simulink model "T1_PreLab_2"  (R2023a)
settings: Solver=VariableStepAuto  StartTime=0.0  StopTime=100  RelTol=1e-3
libraries: dspmathops x30, dspfdesign x15, dspsrcs4 x15, commsink2 x15, dspsigops x15, commrandsrc3 x1
settings Model: Creator=HP VICTUS  LastModifiedBy=HP VICTUS

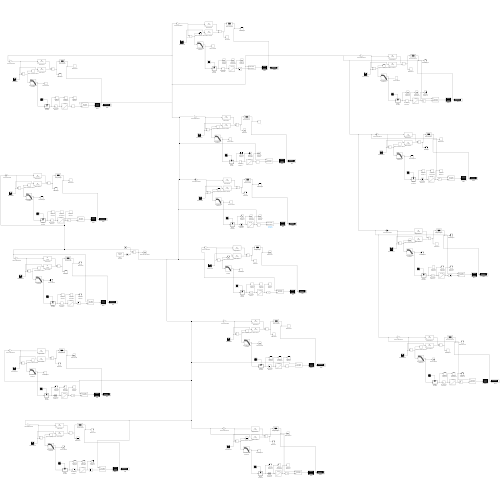
[thumbnail: Simulink's stored preview of the top-level diagram]
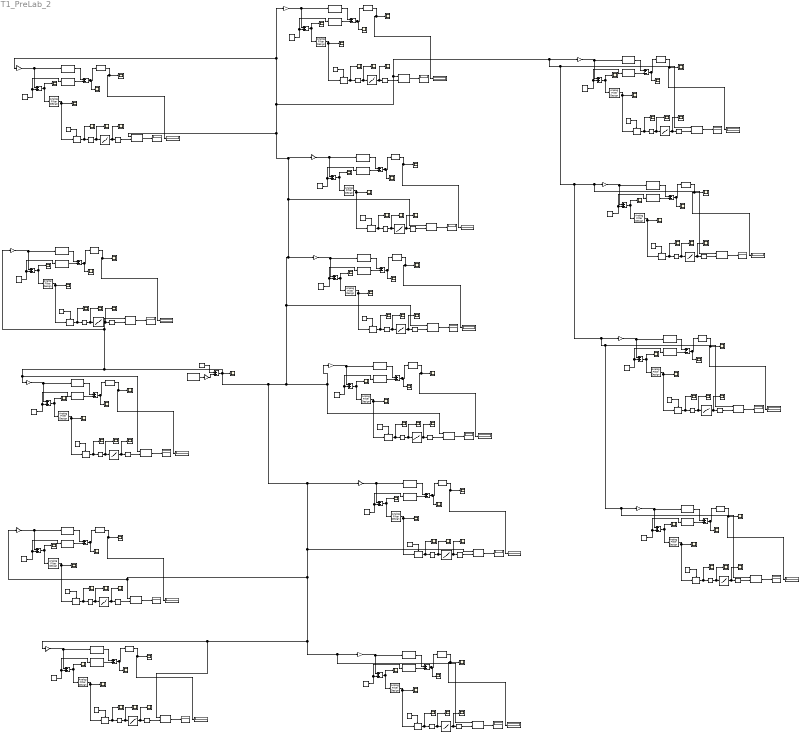
== system T1_PreLab_2 ==
  1-D Lookup Table{,1..14} (15 alike) : Lookup_n-D  NumberOfTableDimensions=1  BreakpointsForDimension1=[-1,1]  Table=[-4,4]  TableDataTypeStr=Inherit: Inherit from 'Table data'  InternalRulePriority=Speed  RndMeth=Simplest
  Add{,1..15} (16 alike) : Sum
  BER{,1..14} (15 alike) : Display
  Binary Generator : commrandsrc3/Bernoulli Binary Generator  ProbabilityOfZero=0.5  SeedSource=Parameter  Seed=61  SampleTime=0.1  SamplesPerFrame=1  OutputDataType=double  SimulateUsing=Interpreted execution
  Channel Attenuation{,1..14} (15 alike) : Gain  Gain=0.5
  Channel Bandwidth Limitation{,1..14} (15 alike) : dspfdesign/Analog Filter Design  method=Butterworth  filttype=Lowpass  N=10  Wlo=1000  Whi=80  Rp=2  Rs=40
  Channel Noise : dspsrcs4/Random Source  SrcType=Gaussian  NormMethod=Ziggurat  CltLength=12  MinVal=0  MaxVal=1  MeanVal=0  VarVal=2  RepMode=Not repeatable  rawSeed=1  IsInherit=off  SampMode=Discrete  SampTime=0.01  SampFrame=1  DataType=Double  OutComplex=Real  OutputFrames=off
  Channel Noise1 : dspsrcs4/Random Source  SrcType=Gaussian  NormMethod=Ziggurat  CltLength=12  MinVal=0  MaxVal=1  MeanVal=0  VarVal=1.6  RepMode=Not repeatable  rawSeed=1  IsInherit=off  SampMode=Discrete  SampTime=0.01  SampFrame=1  DataType=Double  OutComplex=Real  OutputFrames=off
  Channel Noise10 : dspsrcs4/Random Source  SrcType=Gaussian  NormMethod=Ziggurat  CltLength=12  MinVal=0  MaxVal=1  MeanVal=0  VarVal=2.8  RepMode=Not repeatable  rawSeed=1  IsInherit=off  SampMode=Discrete  SampTime=0.01  SampFrame=1  DataType=Double  OutComplex=Real  OutputFrames=off
  Channel Noise11 : dspsrcs4/Random Source  SrcType=Gaussian  NormMethod=Ziggurat  CltLength=12  MinVal=0  MaxVal=1  MeanVal=0  VarVal=2.3  RepMode=Not repeatable  rawSeed=1  IsInherit=off  SampMode=Discrete  SampTime=0.01  SampFrame=1  DataType=Double  OutComplex=Real  OutputFrames=off
  Channel Noise12 : dspsrcs4/Random Source  SrcType=Gaussian  NormMethod=Ziggurat  CltLength=12  MinVal=0  MaxVal=1  MeanVal=0  VarVal=3.5  RepMode=Not repeatable  rawSeed=1  IsInherit=off  SampMode=Discrete  SampTime=0.01  SampFrame=1  DataType=Double  OutComplex=Real  OutputFrames=off
  Channel Noise13 : dspsrcs4/Random Source  SrcType=Gaussian  NormMethod=Ziggurat  CltLength=12  MinVal=0  MaxVal=1  MeanVal=0  VarVal=0.2  RepMode=Not repeatable  rawSeed=1  IsInherit=off  SampMode=Discrete  SampTime=0.01  SampFrame=1  DataType=Double  OutComplex=Real  OutputFrames=off
  Channel Noise14 : dspsrcs4/Random Source  SrcType=Gaussian  NormMethod=Ziggurat  CltLength=12  MinVal=0  MaxVal=1  MeanVal=0  VarVal=0.4  RepMode=Not repeatable  rawSeed=1  IsInherit=off  SampMode=Discrete  SampTime=0.01  SampFrame=1  DataType=Double  OutComplex=Real  OutputFrames=off
  Channel Noise2 : dspsrcs4/Random Source  SrcType=Gaussian  NormMethod=Ziggurat  CltLength=12  MinVal=0  MaxVal=1  MeanVal=0  VarVal=1.9  RepMode=Not repeatable  rawSeed=1  IsInherit=off  SampMode=Discrete  SampTime=0.01  SampFrame=1  DataType=Double  OutComplex=Real  OutputFrames=off
  Channel Noise3 : dspsrcs4/Random Source  SrcType=Gaussian  NormMethod=Ziggurat  CltLength=12  MinVal=0  MaxVal=1  MeanVal=0  VarVal=2.4  RepMode=Not repeatable  rawSeed=1  IsInherit=off  SampMode=Discrete  SampTime=0.01  SampFrame=1  DataType=Double  OutComplex=Real  OutputFrames=off
  Channel Noise4 : dspsrcs4/Random Source  SrcType=Gaussian  NormMethod=Ziggurat  CltLength=12  MinVal=0  MaxVal=1  MeanVal=0  VarVal=0.3  RepMode=Not repeatable  rawSeed=1  IsInherit=off  SampMode=Discrete  SampTime=0.01  SampFrame=1  DataType=Double  OutComplex=Real  OutputFrames=off
  Channel Noise5 : dspsrcs4/Random Source  SrcType=Gaussian  NormMethod=Ziggurat  CltLength=12  MinVal=0  MaxVal=1  MeanVal=0  VarVal=0.5  RepMode=Not repeatable  rawSeed=1  IsInherit=off  SampMode=Discrete  SampTime=0.01  SampFrame=1  DataType=Double  OutComplex=Real  OutputFrames=off
  Channel Noise6 : dspsrcs4/Random Source  SrcType=Gaussian  NormMethod=Ziggurat  CltLength=12  MinVal=0  MaxVal=1  MeanVal=0  VarVal=0.7  RepMode=Not repeatable  rawSeed=1  IsInherit=off  SampMode=Discrete  SampTime=0.01  SampFrame=1  DataType=Double  OutComplex=Real  OutputFrames=off
  Channel Noise7 : dspsrcs4/Random Source  SrcType=Gaussian  NormMethod=Ziggurat  CltLength=12  MinVal=0  MaxVal=1  MeanVal=0  VarVal=0.1  RepMode=Not repeatable  rawSeed=1  IsInherit=off  SampMode=Discrete  SampTime=0.01  SampFrame=1  DataType=Double  OutComplex=Real  OutputFrames=off
  Channel Noise8 : dspsrcs4/Random Source  SrcType=Gaussian  NormMethod=Ziggurat  CltLength=12  MinVal=0  MaxVal=1  MeanVal=0  VarVal=1.3  RepMode=Not repeatable  rawSeed=1  IsInherit=off  SampMode=Discrete  SampTime=0.01  SampFrame=1  DataType=Double  OutComplex=Real  OutputFrames=off
  Channel Noise9 : dspsrcs4/Random Source  SrcType=Gaussian  NormMethod=Ziggurat  CltLength=12  MinVal=0  MaxVal=1  MeanVal=0  VarVal=1  RepMode=Not repeatable  rawSeed=1  IsInherit=off  SampMode=Discrete  SampTime=0.01  SampFrame=1  DataType=Double  OutComplex=Real  OutputFrames=off
  Channel Output{,1..14} (15 alike) : Scope
  Constant : Constant  Value=-4  SampleTime=-1
  Digital Information Signal : Scope
  Error Rate Calculation{,1..14} (15 alike) : commsink2/Error Rate Calculation  N=1  st_delay=0  cp_mode=Entire frame  subframe=[]  PMode=Port  WsName=ErrorVec  RsMode2=off  stop=off  numErr=100  maxBits=1e6
      settings: LibrarySourceBlock=|
      | commhdlsink/Error Rate
      | Calculation
  Gain : Gain  Gain=8
  Moving Average{,1..14} (15 alike) : DiscreteFir  Coefficients=ones(1,1000)/1000  SampleTime=0.001
  Noise  Power{,1..14} (15 alike) : dspmathops/dB Conversion  dBtype=dB  intype=Amplitude  R=1  fuzz=off
      settings: LibrarySourceBlock=commutil2/dB Conversion
  Output from Detector{,1..14} (15 alike) : Scope
  Output from Sampler{,1..14} (15 alike) : Scope
  Output from Thresholder{,1..14} (15 alike) : Scope
  Pulse Generator{,1..14} (15 alike) : DiscretePulseGenerator  PulseType=Time based  Period=0.1  PulseWidth=50
  SNR{,1..14} (15 alike) : Display
  SNR Average{,1..14} (15 alike) : Scope
  SNR Graph{,1..14} (15 alike) : Scope
  Sample and Hold{,1..14} (15 alike) : dspsigops/Sample and Hold  trig=Rising edge  initCond=0  latchinput=off
  Signal Power{,1..14} (15 alike) : dspmathops/dB Conversion  dBtype=dB  intype=Amplitude  R=1  fuzz=off
      settings: LibrarySourceBlock=commutil2/dB Conversion
  Signal corrupted by Noice{,1..14} (15 alike) : Scope
  Subtract{,1..14} (15 alike) : Sum  Inputs=+-
  Zero Crossing Detector{,1..14} (15 alike) : Signum
  Zero-Order Hold{,1..14} (15 alike) : ZeroOrderHold  SampleTime=0.1
  wires:
  Binary Generator/1 -> Gain/1
  Gain/1 -> Add/2
  Constant/1 -> Add/1
  Channel Attenuation/1 -> Add1/1, Signal Power/1
  Channel Noise/1 -> Add1/2, Noise  Power/1
  Add1/1 -> Channel Bandwidth Limitation/1, Signal corrupted by Noice/1
  Channel Bandwidth Limitation/1 -> Sample and Hold/1, Channel Output/1
  Pulse Generator/1 -> Sample and Hold/Trigger
  Error Rate Calculation/1 -> BER/1
  Zero-Order Hold/1 -> Error Rate Calculation/2
  1-D Lookup Table/1 -> Output from Detector/1, Zero-Order Hold/1
  Zero Crossing Detector/1 -> Output from Thresholder/1, 1-D Lookup Table/1
  Sample and Hold/1 -> Output from Sampler/1, Zero Crossing Detector/1
  Moving Average/1 -> SNR/1, SNR Average/1
  Subtract/1 -> SNR Graph/1, Moving Average/1
  Signal Power/1 -> Subtract/1
  Noise  Power/1 -> Subtract/2
  Noise  Power1/1 -> Subtract1/2
  Subtract1/1 -> SNR Graph1/1, Moving Average1/1
  Sample and Hold1/1 -> Output from Sampler1/1, Zero Crossing Detector1/1
  Signal Power1/1 -> Subtract1/1
  Error Rate Calculation1/1 -> BER1/1
  Zero-Order Hold1/1 -> Error Rate Calculation1/2
  Channel Bandwidth Limitation1/1 -> Sample and Hold1/1, Channel Output1/1
  Add2/1 -> Channel Bandwidth Limitation1/1, Signal corrupted by Noice1/1
  Moving Average1/1 -> SNR1/1, SNR Average1/1
  Pulse Generator1/1 -> Sample and Hold1/Trigger
  Channel Attenuation1/1 -> Add2/1, Signal Power1/1
  Channel Noise1/1 -> Add2/2, Noise  Power1/1
  Zero Crossing Detector1/1 -> Output from Thresholder1/1, 1-D Lookup Table1/1
  1-D Lookup Table1/1 -> Output from Detector1/1, Zero-Order Hold1/1
  Noise  Power2/1 -> Subtract2/2
  Subtract2/1 -> SNR Graph2/1, Moving Average2/1
  Sample and Hold2/1 -> Output from Sampler2/1, Zero Crossing Detector2/1
  Signal Power2/1 -> Subtract2/1
  Error Rate Calculation2/1 -> BER2/1
  Zero-Order Hold2/1 -> Error Rate Calculation2/2
  Channel Bandwidth Limitation2/1 -> Sample and Hold2/1, Channel Output2/1
  Add3/1 -> Channel Bandwidth Limitation2/1, Signal corrupted by Noice2/1
  Moving Average2/1 -> SNR2/1, SNR Average2/1
  Pulse Generator2/1 -> Sample and Hold2/Trigger
  Channel Attenuation2/1 -> Add3/1, Signal Power2/1
  Channel Noise2/1 -> Add3/2, Noise  Power2/1
  Zero Crossing Detector2/1 -> Output from Thresholder2/1, 1-D Lookup Table2/1
  1-D Lookup Table2/1 -> Output from Detector2/1, Zero-Order Hold2/1
  Noise  Power3/1 -> Subtract3/2
  Subtract3/1 -> SNR Graph3/1, Moving Average3/1
  Sample and Hold3/1 -> Output from Sampler3/1, Zero Crossing Detector3/1
  Signal Power3/1 -> Subtract3/1
  Error Rate Calculation3/1 -> BER3/1
  Zero-Order Hold3/1 -> Error Rate Calculation3/2
  Channel Bandwidth Limitation3/1 -> Sample and Hold3/1, Channel Output3/1
  Add4/1 -> Channel Bandwidth Limitation3/1, Signal corrupted by Noice3/1
  Moving Average3/1 -> SNR3/1, SNR Average3/1
  Pulse Generator3/1 -> Sample and Hold3/Trigger
  Channel Attenuation3/1 -> Add4/1, Signal Power3/1
  Channel Noise3/1 -> Add4/2, Noise  Power3/1
  Zero Crossing Detector3/1 -> Output from Thresholder3/1, 1-D Lookup Table3/1
  1-D Lookup Table3/1 -> Output from Detector3/1, Zero-Order Hold3/1
  Noise  Power4/1 -> Subtract4/2
  Subtract4/1 -> SNR Graph4/1, Moving Average4/1
  Sample and Hold4/1 -> Output from Sampler4/1, Zero Crossing Detector4/1
  Signal Power4/1 -> Subtract4/1
  Error Rate Calculation4/1 -> BER4/1
  Zero-Order Hold4/1 -> Error Rate Calculation4/2
  Channel Bandwidth Limitation4/1 -> Sample and Hold4/1, Channel Output4/1
  Add5/1 -> Channel Bandwidth Limitation4/1, Signal corrupted by Noice4/1
  Moving Average4/1 -> SNR4/1, SNR Average4/1
  Pulse Generator4/1 -> Sample and Hold4/Trigger
  Channel Attenuation4/1 -> Add5/1, Signal Power4/1
  Channel Noise4/1 -> Add5/2, Noise  Power4/1
  Zero Crossing Detector4/1 -> Output from Thresholder4/1, 1-D Lookup Table4/1
  1-D Lookup Table4/1 -> Output from Detector4/1, Zero-Order Hold4/1
  Noise  Power5/1 -> Subtract5/2
  Subtract5/1 -> SNR Graph5/1, Moving Average5/1
  Sample and Hold5/1 -> Output from Sampler5/1, Zero Crossing Detector5/1
  Signal Power5/1 -> Subtract5/1
  Error Rate Calculation5/1 -> BER5/1
  Zero-Order Hold5/1 -> Error Rate Calculation5/2
  Channel Bandwidth Limitation5/1 -> Sample and Hold5/1, Channel Output5/1
  Add6/1 -> Channel Bandwidth Limitation5/1, Signal corrupted by Noice5/1
  Moving Average5/1 -> SNR5/1, SNR Average5/1
  Pulse Generator5/1 -> Sample and Hold5/Trigger
  Channel Attenuation5/1 -> Add6/1, Signal Power5/1
  Channel Noise5/1 -> Add6/2, Noise  Power5/1
  Zero Crossing Detector5/1 -> Output from Thresholder5/1, 1-D Lookup Table5/1
  1-D Lookup Table5/1 -> Output from Detector5/1, Zero-Order Hold5/1
  Noise  Power6/1 -> Subtract6/2
  Subtract6/1 -> SNR Graph6/1, Moving Average6/1
  Sample and Hold6/1 -> Output from Sampler6/1, Zero Crossing Detector6/1
  Signal Power6/1 -> Subtract6/1
  Error Rate Calculation6/1 -> BER6/1
  Zero-Order Hold6/1 -> Error Rate Calculation6/2
  Channel Bandwidth Limitation6/1 -> Sample and Hold6/1, Channel Output6/1
  Add7/1 -> Channel Bandwidth Limitation6/1, Signal corrupted by Noice6/1
  Moving Average6/1 -> SNR6/1, SNR Average6/1
  Pulse Generator6/1 -> Sample and Hold6/Trigger
  Channel Attenuation6/1 -> Add7/1, Signal Power6/1
  Channel Noise6/1 -> Add7/2, Noise  Power6/1
  Zero Crossing Detector6/1 -> Output from Thresholder6/1, 1-D Lookup Table6/1
  1-D Lookup Table6/1 -> Output from Detector6/1, Zero-Order Hold6/1
  Noise  Power7/1 -> Subtract7/2
  Subtract7/1 -> SNR Graph7/1, Moving Average7/1
  Sample and Hold7/1 -> Output from Sampler7/1, Zero Crossing Detector7/1
  Signal Power7/1 -> Subtract7/1
  Error Rate Calculation7/1 -> BER7/1
  Zero-Order Hold7/1 -> Error Rate Calculation7/2
  Channel Bandwidth Limitation7/1 -> Sample and Hold7/1, Channel Output7/1
  Add8/1 -> Channel Bandwidth Limitation7/1, Signal corrupted by Noice7/1
  Moving Average7/1 -> SNR7/1, SNR Average7/1
  Pulse Generator7/1 -> Sample and Hold7/Trigger
  Channel Attenuation7/1 -> Add8/1, Signal Power7/1
  Channel Noise7/1 -> Add8/2, Noise  Power7/1
  Zero Crossing Detector7/1 -> Output from Thresholder7/1, 1-D Lookup Table7/1
  1-D Lookup Table7/1 -> Output from Detector7/1, Zero-Order Hold7/1
  Noise  Power8/1 -> Subtract8/2
  Subtract8/1 -> SNR Graph8/1, Moving Average8/1
  Sample and Hold8/1 -> Output from Sampler8/1, Zero Crossing Detector8/1
  Signal Power8/1 -> Subtract8/1
  Error Rate Calculation8/1 -> BER8/1
  Zero-Order Hold8/1 -> Error Rate Calculation8/2
  Channel Bandwidth Limitation8/1 -> Sample and Hold8/1, Channel Output8/1
  Add9/1 -> Channel Bandwidth Limitation8/1, Signal corrupted by Noice8/1
  Moving Average8/1 -> SNR8/1, SNR Average8/1
  Pulse Generator8/1 -> Sample and Hold8/Trigger
  Channel Attenuation8/1 -> Add9/1, Signal Power8/1
  Channel Noise8/1 -> Add9/2, Noise  Power8/1
  Zero Crossing Detector8/1 -> Output from Thresholder8/1, 1-D Lookup Table8/1
  1-D Lookup Table8/1 -> Output from Detector8/1, Zero-Order Hold8/1
  Noise  Power9/1 -> Subtract9/2
  Subtract9/1 -> SNR Graph9/1, Moving Average9/1
  Sample and Hold9/1 -> Output from Sampler9/1, Zero Crossing Detector9/1
  Signal Power9/1 -> Subtract9/1
  Error Rate Calculation9/1 -> BER9/1
  Zero-Order Hold9/1 -> Error Rate Calculation9/2
  Channel Bandwidth Limitation9/1 -> Sample and Hold9/1, Channel Output9/1
  Add10/1 -> Channel Bandwidth Limitation9/1, Signal corrupted by Noice9/1
  Moving Average9/1 -> SNR9/1, SNR Average9/1
  Pulse Generator9/1 -> Sample and Hold9/Trigger
  Channel Attenuation9/1 -> Add10/1, Signal Power9/1
  Channel Noise9/1 -> Add10/2, Noise  Power9/1
  Zero Crossing Detector9/1 -> Output from Thresholder9/1, 1-D Lookup Table9/1
  1-D Lookup Table9/1 -> Output from Detector9/1, Zero-Order Hold9/1
  Noise  Power10/1 -> Subtract10/2
  Subtract10/1 -> SNR Graph10/1, Moving Average10/1
  Sample and Hold10/1 -> Output from Sampler10/1, Zero Crossing Detector10/1
  Signal Power10/1 -> Subtract10/1
  Error Rate Calculation10/1 -> BER10/1
  Zero-Order Hold10/1 -> Error Rate Calculation10/2
  Channel Bandwidth Limitation10/1 -> Sample and Hold10/1, Channel Output10/1
  Add11/1 -> Channel Bandwidth Limitation10/1, Signal corrupted by Noice10/1
  Moving Average10/1 -> SNR10/1, SNR Average10/1
  Pulse Generator10/1 -> Sample and Hold10/Trigger
  Channel Attenuation10/1 -> Add11/1, Signal Power10/1
  Channel Noise10/1 -> Add11/2, Noise  Power10/1
  Zero Crossing Detector10/1 -> Output from Thresholder10/1, 1-D Lookup Table10/1
  1-D Lookup Table10/1 -> Output from Detector10/1, Zero-Order Hold10/1
  Noise  Power11/1 -> Subtract11/2
  Subtract11/1 -> SNR Graph11/1, Moving Average11/1
  Sample and Hold11/1 -> Output from Sampler11/1, Zero Crossing Detector11/1
  Signal Power11/1 -> Subtract11/1
  Error Rate Calculation11/1 -> BER11/1
  Zero-Order Hold11/1 -> Error Rate Calculation11/2
  Channel Bandwidth Limitation11/1 -> Sample and Hold11/1, Channel Output11/1
  Add12/1 -> Channel Bandwidth Limitation11/1, Signal corrupted by Noice11/1
  Moving Average11/1 -> SNR11/1, SNR Average11/1
  Pulse Generator11/1 -> Sample and Hold11/Trigger
  Channel Attenuation11/1 -> Add12/1, Signal Power11/1
  Channel Noise11/1 -> Add12/2, Noise  Power11/1
  Zero Crossing Detector11/1 -> Output from Thresholder11/1, 1-D Lookup Table11/1
  1-D Lookup Table11/1 -> Output from Detector11/1, Zero-Order Hold11/1
  Noise  Power12/1 -> Subtract12/2
  Subtract12/1 -> SNR Graph12/1, Moving Average12/1
  Sample and Hold12/1 -> Output from Sampler12/1, Zero Crossing Detector12/1
  Signal Power12/1 -> Subtract12/1
  Error Rate Calculation12/1 -> BER12/1
  Zero-Order Hold12/1 -> Error Rate Calculation12/2
  Channel Bandwidth Limitation12/1 -> Sample and Hold12/1, Channel Output12/1
  Add13/1 -> Channel Bandwidth Limitation12/1, Signal corrupted by Noice12/1
  Moving Average12/1 -> SNR12/1, SNR Average12/1
  Pulse Generator12/1 -> Sample and Hold12/Trigger
  Channel Attenuation12/1 -> Add13/1, Signal Power12/1
  Channel Noise12/1 -> Add13/2, Noise  Power12/1
  Zero Crossing Detector12/1 -> Output from Thresholder12/1, 1-D Lookup Table12/1
  1-D Lookup Table12/1 -> Output from Detector12/1, Zero-Order Hold12/1
  Noise  Power13/1 -> Subtract13/2
  Subtract13/1 -> SNR Graph13/1, Moving Average13/1
  Sample and Hold13/1 -> Output from Sampler13/1, Zero Crossing Detector13/1
  Signal Power13/1 -> Subtract13/1
  Error Rate Calculation13/1 -> BER13/1
  Zero-Order Hold13/1 -> Error Rate Calculation13/2
  Channel Bandwidth Limitation13/1 -> Sample and Hold13/1, Channel Output13/1
  Add14/1 -> Channel Bandwidth Limitation13/1, Signal corrupted by Noice13/1
  Moving Average13/1 -> SNR13/1, SNR Average13/1
  Pulse Generator13/1 -> Sample and Hold13/Trigger
  Channel Attenuation13/1 -> Add14/1, Signal Power13/1
  Channel Noise13/1 -> Add14/2, Noise  Power13/1
  Zero Crossing Detector13/1 -> Output from Thresholder13/1, 1-D Lookup Table13/1
  1-D Lookup Table13/1 -> Output from Detector13/1, Zero-Order Hold13/1
  Noise  Power14/1 -> Subtract14/2
  Subtract14/1 -> SNR Graph14/1, Moving Average14/1
  Sample and Hold14/1 -> Output from Sampler14/1, Zero Crossing Detector14/1
  Signal Power14/1 -> Subtract14/1
  Error Rate Calculation14/1 -> BER14/1
  Zero-Order Hold14/1 -> Error Rate Calculation14/2
  Channel Bandwidth Limitation14/1 -> Sample and Hold14/1, Channel Output14/1
  Add15/1 -> Channel Bandwidth Limitation14/1, Signal corrupted by Noice14/1
  Moving Average14/1 -> SNR14/1, SNR Average14/1
  Pulse Generator14/1 -> Sample and Hold14/Trigger
  Channel Attenuation14/1 -> Add15/1, Signal Power14/1
  Channel Noise14/1 -> Add15/2, Noise  Power14/1
  Zero Crossing Detector14/1 -> Output from Thresholder14/1, 1-D Lookup Table14/1
  1-D Lookup Table14/1 -> Output from Detector14/1, Zero-Order Hold14/1
  Add/1 -> Channel Attenuation3/1, Error Rate Calculation3/1, Channel Attenuation6/1, Error Rate Calculation6/1, Error Rate Calculation9/1, Channel Attenuation9/1, Error Rate Calculation10/1, Channel Attenuation10/1, Error Rate Calculation1/1, Error Rate Calculation7/1, Error Rate Calculation12/1, Channel Attenuation12/1, Error Rate Calculation11/1, Channel Attenuation11/1, Error Rate Calculation13/1, Channel Attenuation13/1, Error Rate Calculation14/1, Channel Attenuation14/1, Error Rate Calculation8/1, Channel Attenuation7/1, Channel Attenuation8/1, Channel Attenuation1/1, Channel Attenuation2/1, Error Rate Calculation2/1, Error Rate Calculation/1, Channel Attenuation/1, Channel Attenuation5/1, Error Rate Calculation5/1, Channel Attenuation4/1, Error Rate Calculation4/1, Digital Information Signal/1
